simulink model "sgMdl_Serial_ReadHeaderLoopback"  (R2024b)
settings: Solver=FixedStepAuto  StartTime=0.0  StopTime=inf  RelTol=1e-3
undefined symbols (not defined in the file): standard
libraries: slrealtimeseriallib x6, speedgoatlib_serial x3
Description:
  | Serial - Read Header Loopback
settings Model: ModifiedByFormat=Speedgoat  Creator=Speedgoat  LastModifiedBy=Speedgoat
settings SolverCC: ConcurrentTasks=on  AlgebraicLoopSolver=TrustRegion  PositivePriorityOrder=on
settings OptimizationCC: BlockReduction=off  OptimizeBlockIOStorage=off
settings DebuggingCC: TasksWithSamePriorityMsg=none  UnconnectedInputMsg=warning  UnconnectedOutputMsg=warning  UnconnectedLineMsg=warning
settings HardwareCC: ProdBitPerLong=64  ProdLongLongMode=on  ProdHWDeviceType=Intel->x86-64 (Linux 64)
settings ModelReferenceCC: EnableRefExpFcnMdlSchedulingChecks=on
settings RTWCC: Description=Speedgoat Real-Time Target Machine  SystemTargetFile=speedgoat.tlc  TemplateMakefile=slrealtime_default_tmf  Toolchain=Simulink Real-Time Toolchain  BuildConfiguration=Faster Runs  TargetLang=C++  GPUComputeCapability=3.5  DLArmComputeVersion=19.05
settings SimulinkRealTimeTargetCC: SubcomponentCodeInterfacePackaging=Reusable function  InstructionSetFMA=off  LogToMDFFile=off  SLRTFileLogMaxRuns=10  UseGCCFastMath=on
settings ConfigComp: CovBoundaryAbsTol=1.0e-5

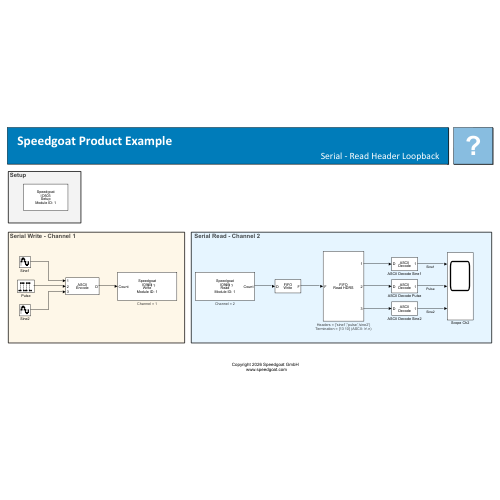
[thumbnail: Simulink's stored preview of the top-level diagram]
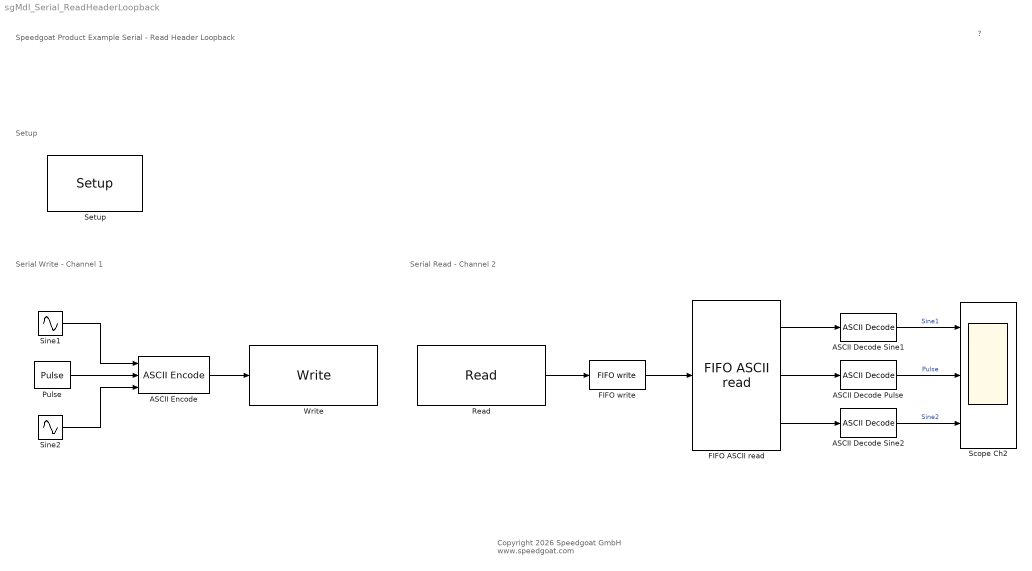
== system sgMdl_Serial_ReadHeaderLoopback ==
  note: Serial Read - Channel 2
  note: Serial Write - Channel 1
  note: Setup
  note: Speedgoat Product Example
      | Serial - Read Header Loopback
  note: ?
  note: Copyright 2026 Speedgoat GmbH
      |  www.speedgoat.com
  ASCII Decode Pulse : slrealtimeseriallib/ASCII Decode  format=pulse %d\r\n  nvars=1  vartypes={ }
  ASCII Decode Sine1 : slrealtimeseriallib/ASCII Decode  format=sine1 %f\r\n  nvars=1  vartypes={'double'}
  ASCII Decode Sine2 : slrealtimeseriallib/ASCII Decode  format=sine2 %f\r\n  nvars=1  vartypes={ }
  ASCII Encode : slrealtimeseriallib/ASCII Encode  format=foo sine1 %f\r\n bar pulse %d\r\n fud sine2 %f\r\n  nvars=3  maxlength=128  vartypes={ 'double' }
  FIFO ASCII read : slrealtimeseriallib/FIFO ASCII read  header={'sine1','pulse','sine2'}  term=[13 10]  hold=Hold last output if no new data  enable=off  maxsize=256  outputtype=8 bit uint null terminated  sampletime=-1
      settings: AttributesFormatString=|
      | Headers = %<header>
      | Termination = %<term> (ASCII: \r\ n)
  FIFO write : slrealtimeseriallib/FIFO write  size=256  inputtype=8 bit uint null terminated  present=off  sampletime=-1  id=FIFO overflow
  Pulse : DiscretePulseGenerator  Period=101  PulseWidth=50  SampleTime=0.01
  "Read " : speedgoatlib_serial/Speedgoat Shared blocks/Read   parModuleType=IO503  parModuleId=1  parChannel=2  parSampleTime=0.01  parFlush=on  parEnLegacy=on  parDataType=8 bit uint null terminated  parSlot=-1  parRxSwFifoSize=128
      settings: AttributesFormatString=Channel = %<parChannel>
  Scope Ch2 : Scope  NumInputPorts=3
  "Setup " : speedgoatlib_serial/Speedgoat Shared blocks/Setup   parModuleType=IO503  parModuleId=1  parSlot=-1  parOscillator=44.2368  parOscillator581=125  parTransceiver1=RS232  parTransceiver2=RS232  parTransceiver3=Disabled  parTransceiver4=Disabled  parTransceiver5=Disabled  parTransceiver6=Disabled  parTransceiver7=Disabled  parTransceiver8=Disabled  parTxTerm1=off  parRxTerm1=off  parMessageMonitoring1=off  parAutoTurnaround1=off  parTurnaroundDelay1=0  parStandardBaud1=on  parBaudrate1=921600  parBaudDivisor1=1  parSamplingRate1=16x (standard)  parPrescale1=None  parCalcBaud1=2764800  parParity1=None  parDataBits1=8  parStopBits1=1  parTxTrigLvl1=1  parRxTrigLvl1=16  parHandshake1=none  parRtsHysteresis1=0  parXon1=17  parXoff1=19  parTxSwFifoSize1=128  parRxSwFifoSize1=128  parTxTerm2=off  parRxTerm2=off  parMessageMonitoring2=off  parAutoTurnaround2=off  parTurnaroundDelay2=0  parStandardBaud2=on  parBaudrate2=921600  parBaudDivisor2=1  parSamplingRate2=16x (standard)  parPrescale2=None  parCalcBaud2=2764800  parParity2=None  parDataBits2=8  parStopBits2=1  parTxTrigLvl2=1  parRxTrigLvl2=16  parHandshake2=none  parRtsHysteresis2=0  parXon2=17  parXoff2=19  parTxSwFifoSize2=128  parRxSwFifoSize2=128  parTxTerm3=off  parRxTerm3=off  parMessageMonitoring3=off  parAutoTurnaround3=off  parTurnaroundDelay3=0  parStandardBaud3=on  parBaudrate3=115200  parBaudDivisor3=1  parSamplingRate3=16x (standard)  parPrescale3=None  parCalcBaud3=2764800  parParity3=None  parDataBits3=8  parStopBits3=1  parTxTrigLvl3=1  parRxTrigLvl3=16  parHandshake3=none  parRtsHysteresis3=0  parXon3=17  parXoff3=19  parTxSwFifoSize3=128  parRxSwFifoSize3=128  parTxTerm4=off  parRxTerm4=off  parMessageMonitoring4=off  parAutoTurnaround4=off  parTurnaroundDelay4=0  parStandardBaud4=on  parBaudrate4=115200  parBaudDivisor4=1  parSamplingRate4=16x (standard)  parPrescale4=None  parCalcBaud4=2764800  parParity4=None  parDataBits4=8  parStopBits4=1  parTxTrigLvl4=1  parRxTrigLvl4=16  parHandshake4=none  parRtsHysteresis4=0  parXon4=17  parXoff4=19  parTxSwFifoSize4=128  parRxSwFifoSize4=128  parTxTerm5=off  parRxTerm5=off  parMessageMonitoring5=off  parAutoTurnaround5=off  parTurnaroundDelay5=0  parStandardBaud5=on  parBaudrate5=115200  parBaudDivisor5=1  parSamplingRate5=16x (standard)  parPrescale5=None  parCalcBaud5=2764800  parParity5=None  parDataBits5=8  parStopBits5=1  parTxTrigLvl5=1  parRxTrigLvl5=1  parHandshake5=none  parRtsHysteresis5=0  parXon5=17  parXoff5=19  parTxSwFifoSize5=1024  parRxSwFifoSize5=1024  parTxTerm6=off  parRxTerm6=off  parMessageMonitoring6=off  parAutoTurnaround6=off  parTurnaroundDelay6=0  parStandardBaud6=on  parBaudrate6=115200  parBaudDivisor6=1  parSamplingRate6=16x (standard)  parPrescale6=None  parCalcBaud6=2764800  parParity6=None  parDataBits6=8  parStopBits6=1  parTxTrigLvl6=1  parRxTrigLvl6=1  parHandshake6=none  parRtsHysteresis6=0  parXon6=17  parXoff6=19  parTxSwFifoSize6=1024  parRxSwFifoSize6=1024  parTxTerm7=off  parRxTerm7=off  parMessageMonitoring7=off  parAutoTurnaround7=off  parTurnaroundDelay7=0  parStandardBaud7=on  parBaudrate7=115200  parBaudDivisor7=1  parSamplingRate7=16x (standard)  parPrescale7=None  parCalcBaud7=2764800  parParity7=None  parDataBits7=8  parStopBits7=1  parTxTrigLvl7=1  parRxTrigLvl7=1  parHandshake7=none  parRtsHysteresis7=0  parXon7=17  parXoff7=19  parTxSwFifoSize7=1024  parRxSwFifoSize7=1024  parTxTerm8=off  parRxTerm8=off  parMessageMonitoring8=off  parAutoTurnaround8=off  parTurnaroundDelay8=0  parStandardBaud8=on  parBaudrate8=115200  parBaudDivisor8=1  parSamplingRate8=16x (standard)  parPrescale8=None  parCalcBaud8=2764800  parParity8=None  parDataBits8=8  parStopBits8=1  parTxTrigLvl8=1  parRxTrigLvl8=1  parHandshake8=none  parRtsHysteresis8=0  parXon8=17  parXoff8=19  parTxSwFifoSize8=1024  parRxSwFifoSize8=1024
  Sine1 : Sin  Amplitude=2  Bias=4  Frequency=10.1  SampleTime=0.01
  Sine2 : Sin  Bias=-2  Frequency=10.11  Phase=3.14  SampleTime=0.01
  "Write " : speedgoatlib_serial/Speedgoat Shared blocks/Write   parModuleType=IO503  parModuleId=1  parChannel=1  parSampleTime=-1  parEnLegacy=on  parDataType=8 bit uint null terminated  parMdlStopMsgEnable=off  parMdlStopMsgData=['CONF' char(13)]  parMdlStopFifoOptions=Write to TX FIFO directly  parMdlStopMsgsDataArr=[67 79 78 70 13]  parMdlStopMsgsDataSize=5  parSlot=-1  parTxSwFifoSize=128
      settings: AttributesFormatString=Channel = %<parChannel>
  wires:
  Sine1/1 -> ASCII Encode/1
  Pulse/1 -> ASCII Encode/2
  Sine2/1 -> ASCII Encode/3
  ASCII Encode/1 -> "Write "/1
  FIFO ASCII read/1 -> ASCII Decode Sine1/1
  FIFO ASCII read/2 -> ASCII Decode Pulse/1
  ASCII Decode Sine1/1 -> Scope Ch2/1  "Sine1"
  FIFO ASCII read/3 -> ASCII Decode Sine2/1
  FIFO write/1 -> FIFO ASCII read/1
  "Read "/1 -> FIFO write/1
  ASCII Decode Pulse/1 -> Scope Ch2/2  "Pulse"
  ASCII Decode Sine2/1 -> Scope Ch2/3  "Sine2"
